simulink model "Tageslichtschaltung"  (R2024b)
settings: Solver=VariableStepAuto  StartTime=0.0  StopTime=24.0  RelTol=1e-3
libraries: simulink x1

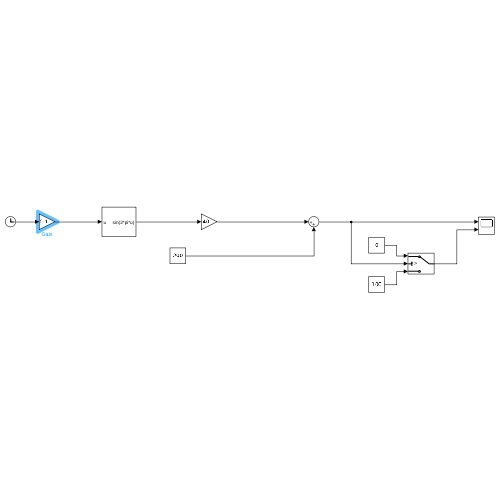
[thumbnail: Simulink's stored preview of the top-level diagram]
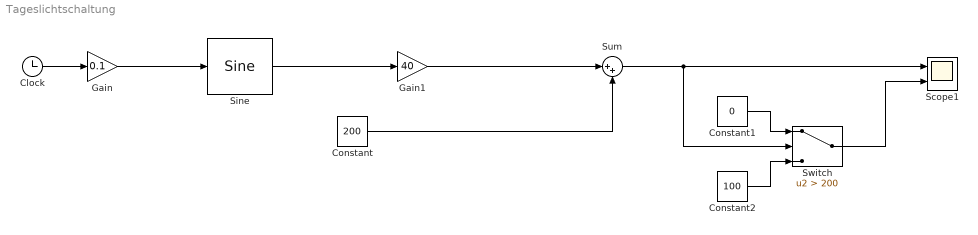
== system Tageslichtschaltung ==
  Clock : Clock
  Constant : Constant  Value=200
  Constant1 : Constant  Value=0
  Constant2 : Constant  Value=100
  Gain : Gain  Gain=0.1
  Gain1 : Gain  Gain=40
  Scope1 : Scope  NumInputPorts=2
  Sine : simulink/Lookup Tables/Sine  Formula=sin(2*pi*u)  NumDataPoints=(2^5)+1  OutputWordLength=16  InternalRulePriority=Speed
  Sum : Sum  Inputs=|++
  Switch : Switch  Criteria=u2 > Threshold  Threshold=200  SaturateOnIntegerOverflow=off  InputSameDT=off
  wires:
  Sine/1 -> Gain1/1
  Constant/1 -> Sum/2
  Clock/1 -> Gain/1
  Gain/1 -> Sine/1
  Gain1/1 -> Sum/1
  Sum/1 -> Switch/2, Scope1/1
  Constant2/1 -> Switch/3
  Constant1/1 -> Switch/1
  Switch/1 -> Scope1/2
